simulink library "INT_T50_VD"  (R2016b)
settings: Solver=VariableStepAuto  StartTime=0.0  StopTime=10.0  RelTol=1e-3
settings Model: Creator=xuxingpei  LastModifiedBy=xuxingpei

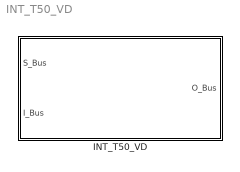
== system INT_T50_VD ==
  INT_T50_VD : Subsystem

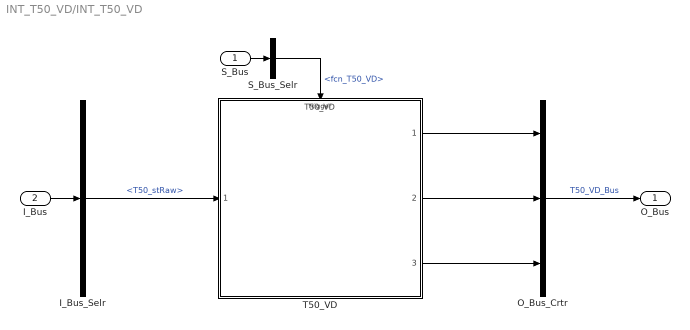
== system INT_T50_VD/INT_T50_VD ==
  S_Bus : Inport
  I_Bus : Inport  Port=2
  I_Bus_Selr : BusSelector  OutputSignals=T50_stRaw
  O_Bus_Crtr : BusCreator  Inputs=3
  S_Bus_Selr : BusSelector  OutputSignals=fcn_T50_VD
  T50_VD : ModelReference  ModelNameDialog=T50_VD  SimulationMode=Normal  ModelReferenceVersion=1.58  TriggerPortName=function  TriggerPortTriggerType=function-call  TriggerPortStatesWhenEnabling=held
  O_Bus : Outport
  wires:
  S_Bus_Selr/1 -> T50_VD/Trigger  "<fcn_T50_VD>"
  S_Bus/1 -> S_Bus_Selr/1
  I_Bus/1 -> I_Bus_Selr/1
  I_Bus_Selr/1 -> T50_VD/1  "<T50_stRaw>"
  O_Bus_Crtr/1 -> O_Bus/1  "T50_VD_Bus"
  T50_VD/1 -> O_Bus_Crtr/1
  T50_VD/2 -> O_Bus_Crtr/2
  T50_VD/3 -> O_Bus_Crtr/3
